simulink model "control"  (R2021b)
settings: Solver=FixedStepDiscrete  StartTime=0.0  StopTime=inf  FixedStep=0.02  RelTol=1e-3
libraries: dspstat3 x1
settings Model: Creator=jekyll  LastModifiedBy=jekyll
settings OptimizationCC: DefaultParameterBehavior=Inlined  EnhancedBackFolding=on  PassReuseOutputArgsAs=Individual arguments  ZeroExternalMemoryAtStartup=off  ZeroInternalMemoryAtStartup=off  OptimizeBlockOrder=speed  DifferentSizesBufferReuse=on  OptimizationCustomize=off  EfficientTunableParamExpr=on
settings DebuggingCC: ParameterTunabilityLossMsg=error  UnconnectedInputMsg=none  UnconnectedOutputMsg=none  UnconnectedLineMsg=none
settings ModelReferenceCC: EnableRefExpFcnMdlSchedulingChecks=off
settings SFSimCC: MATLABDynamicMemAlloc=off
settings RTWCC: Description=Embedded Coder  SystemTargetFile=ert.tlc  GenCodeOnly=on  TemplateMakefile=ert_default_tmf  CustomHeaderCode=#include <emscripten/emscripten.h>  GPUComputeCapability=5.0  DLArmComputeVersion=20.02.1
settings CodeAppCC: ForceParamTrailComments=on  IgnoreCustomStorageClasses=off  OperatorAnnotations=on  SimulinkDataObjDesc=on  SFDataObjDesc=on  InsertBlockDesc=on
settings ERTTargetCC: TargetLangStandard=C99 (ISO)  GenerateSampleERTMain=on  InlinedParameterPlacement=NonHierarchical  ERTCustomFileTemplate=example_file_process.tlc

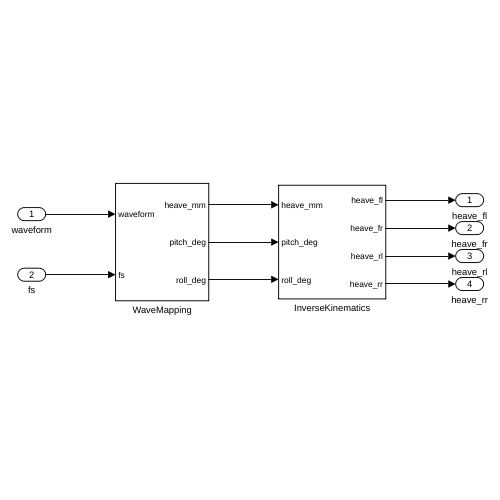
[thumbnail: Simulink's stored preview of the top-level diagram]
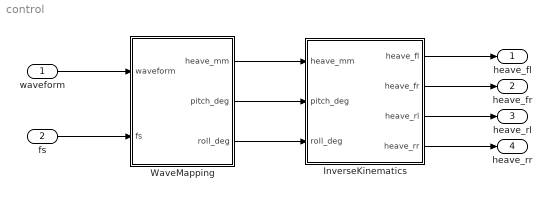
== system control ==
  waveform : Inport  PortDimensions=512
  fs : Inport  Port=2
  InverseKinematics : Subsystem
  WaveMapping : Subsystem
  heave_fl : Outport
  heave_fr : Outport  Port=2
  heave_rl : Outport  Port=3
  heave_rr : Outport  Port=4
  wires:
  fs/1 -> WaveMapping/2(fs)
  WaveMapping/3(roll_deg) -> InverseKinematics/3(roll_deg)
  InverseKinematics/1(heave_fl) -> heave_fl/1
  InverseKinematics/2(heave_fr) -> heave_fr/1
  InverseKinematics/3(heave_rl) -> heave_rl/1
  InverseKinematics/4(heave_rr) -> heave_rr/1
  WaveMapping/1(heave_mm) -> InverseKinematics/1(heave_mm)
  WaveMapping/2(pitch_deg) -> InverseKinematics/2(pitch_deg)
  waveform/1 -> WaveMapping/1(waveform)

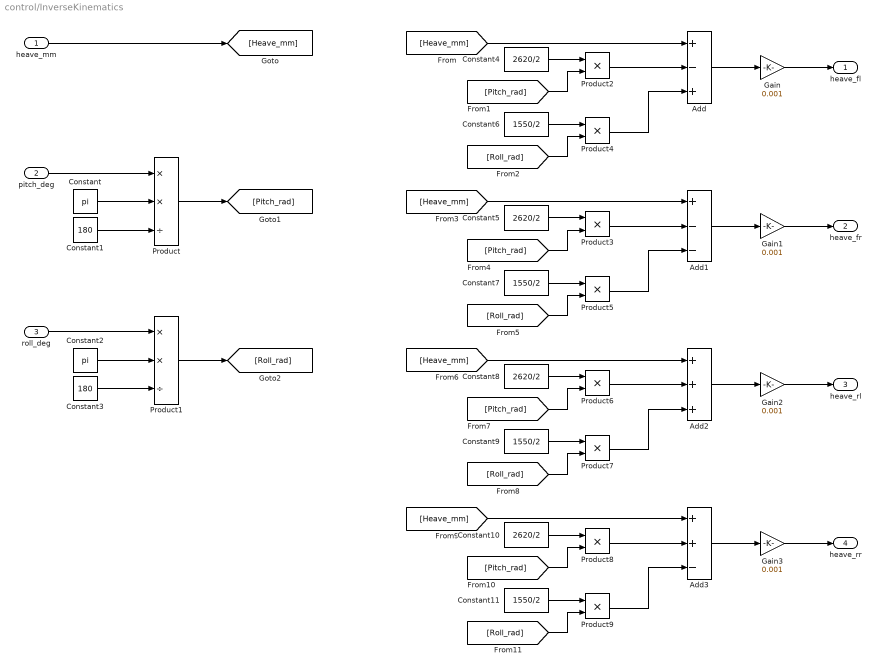
== system control/InverseKinematics ==
  heave_mm : Inport
  pitch_deg : Inport  Port=2
  roll_deg : Inport  Port=3
  Add : Sum  Inputs=+-+
  Add1 : Sum  Inputs=+--
  Add2 : Sum  Inputs=+++
  Add3 : Sum  Inputs=++-
  Constant : Constant  Value=pi
  Constant1 : Constant  Value=180
  Constant{4..5,8,10} (4 alike) : Constant  Value=2620/2
  Constant{6..7,9,11} (4 alike) : Constant  Value=1550/2
  Constant2 : Constant  Value=pi
  Constant3 : Constant  Value=180
  Gain{,1..3} (4 alike) : Gain  Gain=0.001
  Product : Product  Inputs=**/
  Product1 : Product  Inputs=**/
  Product{2..9} (8 alike) : Product
  heave_fl : Outport
  heave_fr : Outport  Port=2
  heave_rl : Outport  Port=3
  heave_rr : Outport  Port=4
  wires:
  Add/1 -> Gain/1
  pitch_deg/1 -> Product/1
  Constant/1 -> Product/2
  Constant1/1 -> Product/3
  Constant3/1 -> Product1/3
  Constant2/1 -> Product1/2
  roll_deg/1 -> Product1/1
  heave_mm/1 -> [Heave_mm]
  Product/1 -> [Pitch_rad]
  Product1/1 -> [Roll_rad]
  [Heave_mm] -> Add/1
  Product2/1 -> Add/2
  Constant4/1 -> Product2/1
  [Pitch_rad] -> Product2/2
  [Roll_rad] -> Product4/2
  Product4/1 -> Add/3
  Constant6/1 -> Product4/1
  Constant7/1 -> Product5/1
  Product5/1 -> Add1/3
  [Roll_rad] -> Product5/2
  [Pitch_rad] -> Product3/2
  Constant5/1 -> Product3/1
  Product3/1 -> Add1/2
  [Heave_mm] -> Add1/1
  Add1/1 -> Gain1/1
  Add2/1 -> Gain2/1
  [Heave_mm] -> Add2/1
  Product6/1 -> Add2/2
  Constant8/1 -> Product6/1
  [Pitch_rad] -> Product6/2
  [Roll_rad] -> Product7/2
  Product7/1 -> Add2/3
  Constant9/1 -> Product7/1
  Constant11/1 -> Product9/1
  Product9/1 -> Add3/3
  [Roll_rad] -> Product9/2
  [Pitch_rad] -> Product8/2
  Constant10/1 -> Product8/1
  Product8/1 -> Add3/2
  [Heave_mm] -> Add3/1
  Add3/1 -> Gain3/1
  Gain/1 -> heave_fl/1
  Gain1/1 -> heave_fr/1
  Gain2/1 -> heave_rl/1
  Gain3/1 -> heave_rr/1

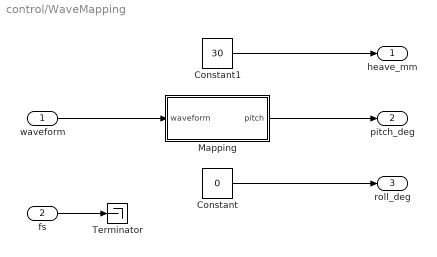
== system control/WaveMapping ==
  waveform : Inport
  fs : Inport  Port=2
  Constant : Constant  Value=0
  Constant1 : Constant  Value=30
  Mapping : Subsystem
  Terminator : Terminator
  heave_mm : Outport
  pitch_deg : Outport  Port=2
  roll_deg : Outport  Port=3
  wires:
  waveform/1 -> Mapping/1(waveform)
  Constant1/1 -> heave_mm/1
  Mapping/1(pitch) -> pitch_deg/1
  fs/1 -> Terminator/1
  Constant/1 -> roll_deg/1

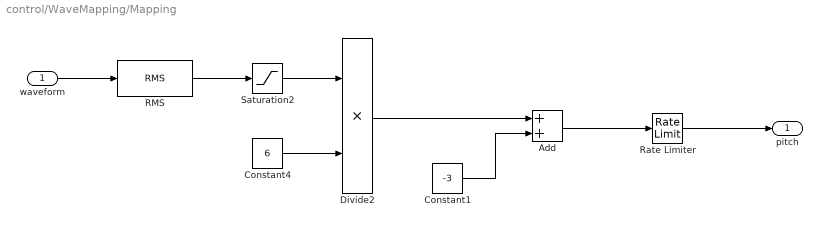
== system control/WaveMapping/Mapping ==
  waveform : Inport
  Add : Sum
  Constant1 : Constant  Value=-3
  Constant4 : Constant  Value=6
  Divide2 : Product  Inputs=**
  RMS : dspstat3/RMS  run=off  directionMode=Entire input  dimension=1  InputProcessing=Columns as channels (frame based)  reset_popup=None
  Rate Limiter : RateLimiter  RisingSlewLimit=3/1  FallingSlewLimit=-3/1  SampleTimeMode=inherited
  Saturation2 : Saturate  UpperLimit=1  LowerLimit=0
  pitch : Outport
  wires:
  Rate Limiter/1 -> pitch/1
  RMS/1 -> Saturation2/1
  waveform/1 -> RMS/1
  Constant4/1 -> Divide2/2
  Add/1 -> Rate Limiter/1
  Saturation2/1 -> Divide2/1
  Divide2/1 -> Add/1
  Constant1/1 -> Add/2
